simulink model "q1_model"  (R2018a)
settings: Solver=VariableStepAuto  StartTime=0.0  StopTime=t_f  FixedStep=dt  RelTol=1e-3
values from neighbouring files (symbols this model uses):
  A = [100  0  0  -57.735026919; 0  100  0  -57.735026919; 0  0  100  -57.735026919]    [data.mat]    (also in q1.m = [h1_hat h2_hat h3_hat h4_hat])
  I_b = [100 1 2; 1 150 3; 2 3 200]    [q1.m]    (also in q3.m)
  Kd = -4    [q1.m]
  omega_B_N_t0 = zeros(3,1)    [q1.m]
libraries: vrlib x1
settings Model: Creator=Padraig Lysandrou  LastModifiedBy=Padraig Lysandrou

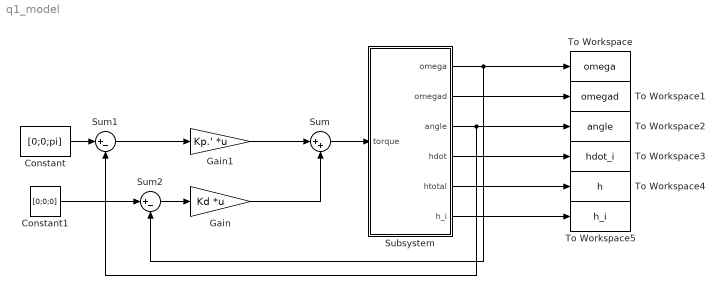
== system q1_model ==
  Constant : Constant  Value=[0;0;pi]
  Constant1 : Constant  Value=[0;0;0]
  Gain : Gain  Gain=Kd  Multiplication=Matrix(K*u) (u vector)
  Gain1 : Gain  Gain=Kp.'  Multiplication=Matrix(K*u) (u vector)
  Subsystem : Subsystem
  Sum : Sum  Inputs=|++
  Sum1 : Sum  Inputs=|+-
  Sum2 : Sum  Inputs=|+-
  To Workspace : ToWorkspace  VariableName=omega  SaveFormat=Timeseries  SampleTime=-1
  To Workspace1 : ToWorkspace  VariableName=omegad  SaveFormat=Timeseries  SampleTime=-1
  To Workspace2 : ToWorkspace  VariableName=angle  SaveFormat=Timeseries  SampleTime=-1
  To Workspace3 : ToWorkspace  VariableName=hdot_i  SaveFormat=Timeseries  SampleTime=-1
  To Workspace4 : ToWorkspace  VariableName=h  SaveFormat=Timeseries  SampleTime=-1
  To Workspace5 : ToWorkspace  VariableName=h_i  SaveFormat=Timeseries  SampleTime=-1
  wires:
  Sum/1 -> Subsystem/1(torque)
  Subsystem/1("omega ") -> Sum2/2, To Workspace/1
  Subsystem/2(omegad) -> To Workspace1/1
  Gain1/1 -> Sum/1
  Gain/1 -> Sum/2
  Sum1/1 -> Gain1/1
  Constant/1 -> Sum1/1
  Subsystem/3(angle) -> Sum1/2, To Workspace2/1
  Constant1/1 -> Sum2/1
  Sum2/1 -> Gain/1
  Subsystem/4(hdot) -> To Workspace3/1
  Subsystem/5(htotal) -> To Workspace4/1
  Subsystem/6(h_i) -> To Workspace5/1

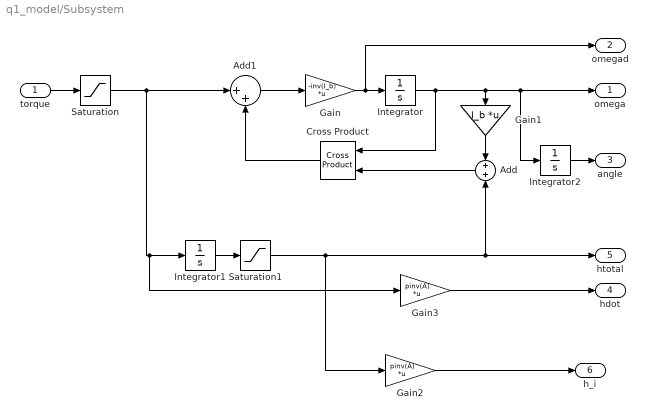
== system q1_model/Subsystem ==
  torque : Inport
  Add : Sum
  Add1 : Sum  Inputs=|++
  Cross Product : vrlib/Utilities/Cross Product
      settings: SourceProductBaseCode=VR
  Gain : Gain  Gain=-inv(I_b)  Multiplication=Matrix(K*u) (u vector)
  Gain1 : Gain  Gain=I_b  Multiplication=Matrix(K*u) (u vector)
  Gain2 : Gain  Gain=pinv(A)  Multiplication=Matrix(K*u) (u vector)
  Gain3 : Gain  Gain=pinv(A)  Multiplication=Matrix(K*u) (u vector)
  Integrator : Integrator  InitialCondition=omega_B_N_t0
  Integrator1 : Integrator  InitialCondition=zeros(3,1)
  Integrator2 : Integrator  InitialCondition=[0;0;0]
  Saturation : Saturate  UpperLimit=0.0002  LowerLimit=-0.0002
  Saturation1 : Saturate  UpperLimit=0.0087  LowerLimit=-0.0087
  "omega " : Outport
  omegad : Outport  Port=2
  angle : Outport  Port=3
  hdot : Outport  Port=4
  htotal : Outport  Port=5
  h_i : Outport  Port=6
  wires:
  Integrator/1 -> Integrator2/1, "omega "/1, Gain1/1, Cross Product/1
  Gain/1 -> omegad/1, Integrator/1
  Gain1/1 -> Add/1
  Add/1 -> Cross Product/2
  Add1/1 -> Gain/1
  Cross Product/1 -> Add1/2
  torque/1 -> Saturation/1
  Saturation/1 -> Add1/1, Gain3/1, Integrator1/1
  Integrator1/1 -> Saturation1/1
  Saturation1/1 -> Gain2/1, Add/2, htotal/1
  Integrator2/1 -> angle/1
  Gain2/1 -> h_i/1
  Gain3/1 -> hdot/1
